simulink model "rtlab_simpowersystems_continuous"  (Simulink 7.8)
settings: Solver=ode3  StartTime=0.0  StopTime=Inf  FixedStep=1e-5  RelTol=1e-3
libraries: powerlib x5, rtlab x2, simulink x1, powerlib_extras x1
Description:
  | Model of a simple control system for use iin training.
settings Model: Creator=Paul Baracos  LastModifiedBy=sfrank1  BufferReuse=off
settings DataIOCC: SaveOutput=off  SaveTime=off  SignalLoggingName=sigsOut
settings OptimizationCC: BlockReduction=off  BooleanDataType=off  InlineInvariantSignals=on  OptimizeBlockIOStorage=off  BufferReuse=off  ExpressionFolding=off  LocalBlockOutputs=off  InitFltsAndDblsToZero=on
settings DebuggingCC: SaveWithParameterizedLinksMsg=none  SignalResolutionControl=TryResolveAllWithWarning  SolverPrmCheckMsg=none  MultiTaskDSMMsg=warning  MultiTaskCondExecSysMsg=none  FcnCallInpInsideContextMsg=Use local settings  StrictBusMsg=None
settings HardwareCC: TargetUnknown=on
settings RTWCC: IncludeERTFirstTime=on
settings GRTTargetCC: TargetFcnLib=ansi_tfl_tmw.mat

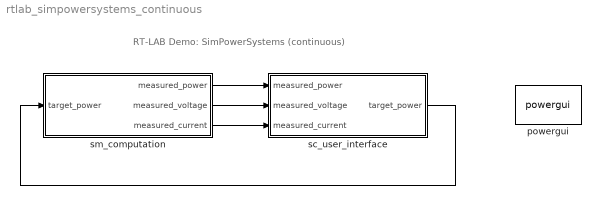
== system rtlab_simpowersystems_continuous ==
  note: RT-LAB Demo: SimPowerSystems (continuous)
  powergui : powerlib/powergui  Priority=1  SimulationMode=Continuous  SolverType=Tustin  SampleTime=50e-6  frequency=60  SPID=off  DisableSnubberDevices=off  DisableRonSwitches=off  DisableVfSwitches=off  SwTol=0  Interpol=off  DisplayEquations=off  FunctionMessages=off  frequencyindice=60  Pbase=100e6  ErrMax=1e-4  Iterations=50  UnitsV=kV  UnitsW=MW  echomessages=off  HookPort=off  EnableUseOfTLC=off  x0status=blocks  RestoreLinks=warning  ResistiveCurrentMeasurement=off  Ylog=off  Xlog=on  ShowGrid=off  save=off  variable=ZData  ZoomFFT=off  StartTime=0.0  cycles=1  DisplayStyle=1  FreqAxis=off  MaxFrequency=1000  frequencyindicesteady=1  display=off  methode=off
  sc_user_interface : Subsystem
  sm_computation : Subsystem
  wires:
  sc_user_interface/1(target_power) -> sm_computation/1(target_power)
  sm_computation/1(measured_power) -> sc_user_interface/1(measured_power)
  sm_computation/2(measured_voltage) -> sc_user_interface/2(measured_voltage)
  sm_computation/3(measured_current) -> sc_user_interface/3(measured_current)

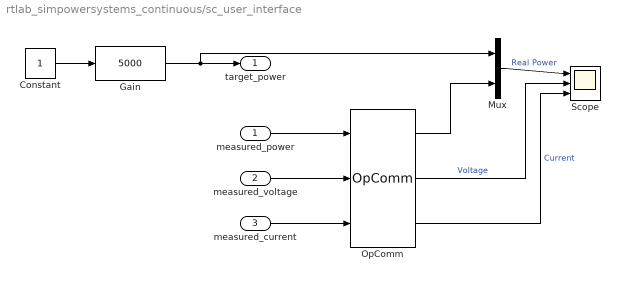
== system rtlab_simpowersystems_continuous/sc_user_interface ==
  measured_power : Inport
  measured_voltage : Inport  Port=2
  measured_current : Inport  Port=3
  Constant : Constant
  Gain : simulink/Math Operations/Slider Gain  low=0  gain=5000  high=20000
  Mux : Mux  Inputs=2
  OpComm : rtlab/OpComm  nbport=3  groupe_acq=1  subsys_rate=0  st=0  Synchronization=on  Interpolation=on  Threshold=1.0  Missed_Data=off  Sim_Time=off  Samples=off  dynSigOut=off  from_console=0  warning_done=off  writeOpCommFile=off  Offset=off
  Scope : Scope  NumInputPorts=3
      settings: YMin=0~-400~-20  YMax=12000~400~20  MaxDataPoints=100000
  target_power : Outport
  wires:
  Gain/1 -> target_power/1, Mux/1
  Mux/1 -> Scope/1  "Real Power"
  measured_power/1 -> OpComm/1
  OpComm/1 -> Mux/2
  Constant/1 -> Gain/1
  measured_current/1 -> OpComm/3
  measured_voltage/1 -> OpComm/2
  OpComm/2 -> Scope/2  "Voltage"
  OpComm/3 -> Scope/3  "Current"

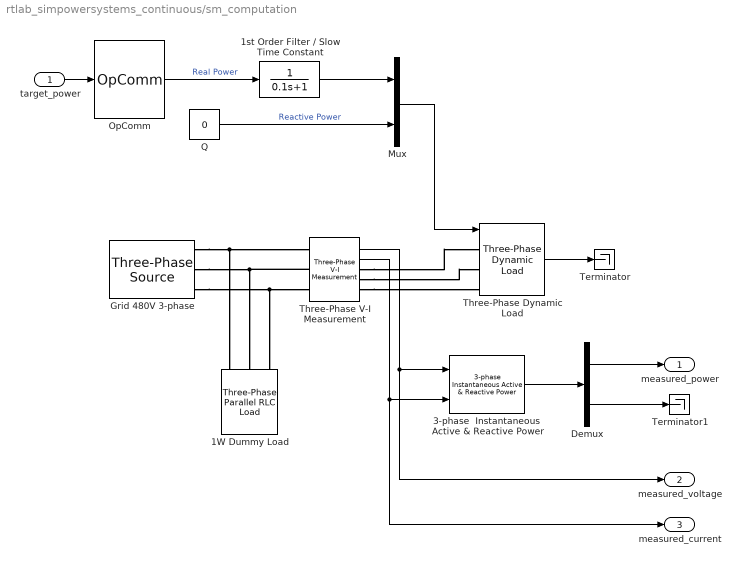
== system rtlab_simpowersystems_continuous/sm_computation ==
  target_power : Inport
  1W Dummy Load : powerlib/Elements/Three-Phase Parallel RLC Load  LConnTagsString=A|B|C  Configuration=Y (grounded)  NominalVoltage=480  NominalFrequency=60  ActivePower=1  InductivePower=0  CapacitivePower=0  Measurements=None  LoadType=constant Z
  1st Order Filter / Slow Time Constant : TransferFcn  Denominator=[0.1 1]
  3-phase  Instantaneous  Active & Reactive Power : powerlib_extras/Measurements/3-phase  Instantaneous  Active & Reactive Power
  Demux : Demux  Outputs=2
  Grid 480V 3-phase : powerlib/Electrical Sources/Three-Phase Source  Voltage=480  PhaseAngle=0  Frequency=60  InternalConnection=Yg  SpecifyImpedance=off  Resistance=0  Inductance=0  ShortCircuitLevel=100e6  BaseVoltage=480  XRratio=7  BusType=swing  Pref=0  Qref=0  Qmin=-inf  Qmax=inf
  Mux : Mux  Inputs=2
  OpComm : rtlab/OpComm  nbport=1  groupe_acq=1  subsys_rate=0  st=0  Synchronization=on  Interpolation=on  Threshold=1.0  Missed_Data=off  Sim_Time=off  Samples=off  dynSigOut=off  from_console=1  warning_done=off  writeOpCommFile=off  Offset=off
  Q : Constant  Value=0
  Terminator : Terminator
  Terminator1 : Terminator
  Three-Phase Dynamic Load : powerlib/Elements/Three-Phase Dynamic Load  NominalVoltage=[480 60]  ActiveReactivePowers=[0 0]  PositiveSequence=[1 0]  ExternalControl=on  NpNq=[1.3 2]  TimeConstants="[0  0  0  0]"  MinimumVoltage=0.7  LoadFlowParameters=[4,0,0,0,0]
  Three-Phase V-I Measurement : powerlib/Measurements/Three-Phase V-I Measurement  VoltageMeasurement=phase-to-ground  SetLabelV=off  LabelV=Vabc  Vpu=off  VpuLL=off  CurrentMeasurement=yes  SetLabelI=off  LabelI=Iabc  Ipu=off  Pbase=100e6  Vbase=500e3  OutputType=Complex  PhasorSimulation=off  PSBequivalent=0
  measured_power : Outport
  measured_voltage : Outport  Port=2
  measured_current : Outport  Port=3
  wires:
  target_power/1 -> OpComm/1
  Three-Phase Dynamic Load/1 -> Terminator/1
  Q/1 -> Mux/2  "Reactive Power"
  3-phase  Instantaneous  Active & Reactive Power/1 -> Demux/1
  Demux/1 -> measured_power/1
  Demux/2 -> Terminator1/1
  Three-Phase V-I Measurement/1 -> measured_voltage/1, 3-phase  Instantaneous  Active & Reactive Power/1
  Three-Phase V-I Measurement/2 -> measured_current/1, 3-phase  Instantaneous  Active & Reactive Power/2
  OpComm/1 -> 1st Order Filter / Slow Time Constant/1  "Real Power"
  1st Order Filter / Slow Time Constant/1 -> Mux/1
  Mux/1 -> Three-Phase Dynamic Load/1
  connections:
  Grid 480V 3-phase/RConn1 -- Three-Phase V-I Measurement/LConn1 -- 1W Dummy Load/LConn1
  Three-Phase V-I Measurement/LConn2 -- Grid 480V 3-phase/RConn2 -- 1W Dummy Load/LConn2
  Grid 480V 3-phase/RConn3 -- Three-Phase V-I Measurement/LConn3 -- 1W Dummy Load/LConn3
  Three-Phase V-I Measurement/RConn1 -- Three-Phase Dynamic Load/LConn1
  Three-Phase V-I Measurement/RConn3 -- Three-Phase Dynamic Load/LConn3
  Three-Phase V-I Measurement/RConn2 -- Three-Phase Dynamic Load/LConn2
